simulink model "threeTetCtrllr_th"  (R2018b)
settings: Solver=VariableStepAuto  StartTime=0.0  StopTime=1  RelTol=1e-3
values from neighbouring files (symbols this model uses):
  alti_sp = 0    [threeTetCtrllr_ts.m]
  eulerAng = [0;0;0]*pi/180    [threeTetCtrllr_ts.m]
  flow = [0;0;0]    [threeTetCtrllr_ts.m]
  OwB = [0;0;0]    [threeTetCtrllr_ts.m]
  pitch_sp = 1*pi/180    (= 0.0174532925199)    [threeTetCtrllr_ts.m]
  Rcm_o = [0;0;0]    [threeTetCtrllr_ts.m]
  roll_sp = 0*pi/180    (= 0)    [threeTetCtrllr_ts.m]
  Vcm_o = zeros(3,1)    [threeTetCtrllr_ts.m]
  yaw_sp = 0*pi/180    (= 0)    [threeTetCtrllr_ts.m]
libraries: threeTetCtrllr_ul x1
settings Model: Creator=Ayaz  LastModifiedBy=asiddiq2

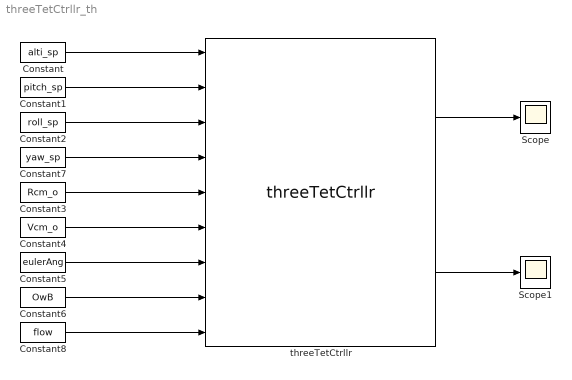
== system threeTetCtrllr_th ==
  Constant : Constant  Value=alti_sp  VectorParams1D=off
  Constant1 : Constant  Value=pitch_sp  VectorParams1D=off
  Constant2 : Constant  Value=roll_sp  VectorParams1D=off
  Constant3 : Constant  Value=Rcm_o  VectorParams1D=off
  Constant4 : Constant  Value=Vcm_o  VectorParams1D=off
  Constant5 : Constant  Value=eulerAng  VectorParams1D=off
  Constant6 : Constant  Value=OwB  VectorParams1D=off
  Constant7 : Constant  Value=yaw_sp  VectorParams1D=off
  Constant8 : Constant  Value=flow  VectorParams1D=off
  Scope : Scope
  Scope1 : Scope
  threeTetCtrllr : threeTetCtrllr_ul/threeTetCtrllr  SystemSampleTime=-1
  wires:
  Constant/1 -> threeTetCtrllr/1
  Constant1/1 -> threeTetCtrllr/2
  Constant2/1 -> threeTetCtrllr/3
  Constant3/1 -> threeTetCtrllr/5
  Constant4/1 -> threeTetCtrllr/6
  Constant5/1 -> threeTetCtrllr/7
  Constant6/1 -> threeTetCtrllr/8
  Constant8/1 -> threeTetCtrllr/9
  threeTetCtrllr/1 -> Scope/1
  threeTetCtrllr/2 -> Scope1/1
  Constant7/1 -> threeTetCtrllr/4
